simulink model "ESTS_FRIC_SLIP2_test"  (R2024b)
settings: Solver=VariableStepAuto  StartTime=0.0  StopTime=10.0  RelTol=1e-3
libraries: ESTS_FRIC_SLIP2 x1
settings Model: Creator=blatak  LastModifiedBy=blatak

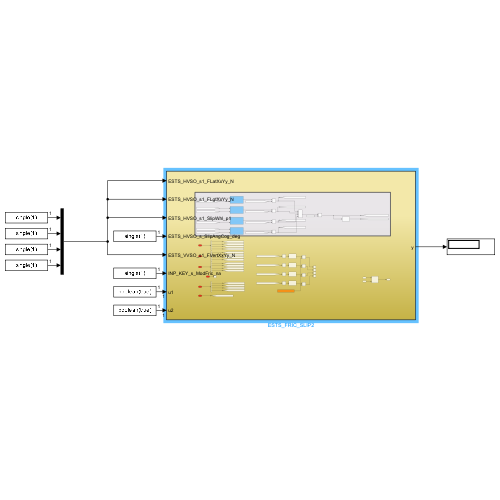
[thumbnail: Simulink's stored preview of the top-level diagram]
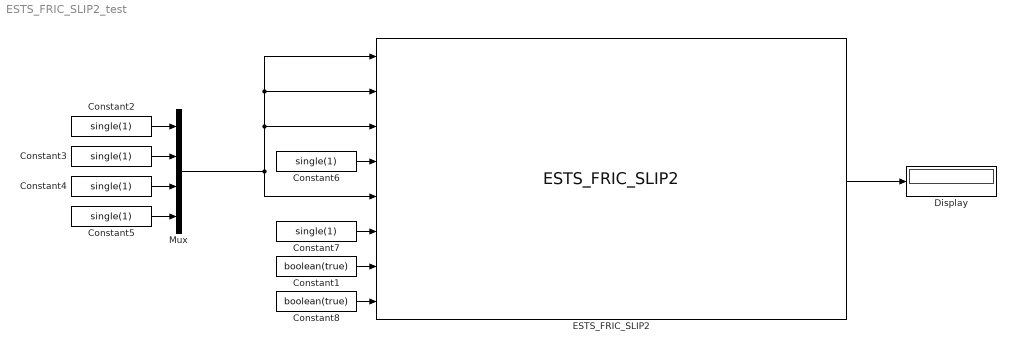
== system ESTS_FRIC_SLIP2_test ==
  Constant1 : Constant  Value=boolean(true)
  Constant{2..7} (6 alike) : Constant  Value=single(1)
  Constant8 : Constant  Value=boolean(true)
  Display : Display
  ESTS_FRIC_SLIP2 : ESTS_FRIC_SLIP2/ESTS_FRIC_SLIP2  SystemSampleTime=-1  VariantActivationTime=update diagram  AllowFlexibleInterface=on  Latency=0  AutoFrameSizeCalculation=off
  Mux : Mux
  wires:
  Constant7/1 -> ESTS_FRIC_SLIP2/6
  Constant4/1 -> Mux/3
  Constant6/1 -> ESTS_FRIC_SLIP2/4
  Constant5/1 -> Mux/4
  Mux/1 -> ESTS_FRIC_SLIP2/5, ESTS_FRIC_SLIP2/3, ESTS_FRIC_SLIP2/2, ESTS_FRIC_SLIP2/1
  Constant3/1 -> Mux/2
  Constant2/1 -> Mux/1
  ESTS_FRIC_SLIP2/1 -> Display/1
  Constant1/1 -> ESTS_FRIC_SLIP2/7
  Constant8/1 -> ESTS_FRIC_SLIP2/8
